simulink model "WaterTank"  (R2025b)
settings: Solver=ode4  StartTime=0.0  StopTime=60  FixedStep=0.01  RelTol=1e-3
InitFcn:
  | WaterTank_script;
undefined symbols (not defined in the file or in its folder): DiscIntNeverNeededParam
libraries: simulink x3, slpidlib x1, rllib x1
settings Model: Creator=Administrator  LastModifiedBy=chang

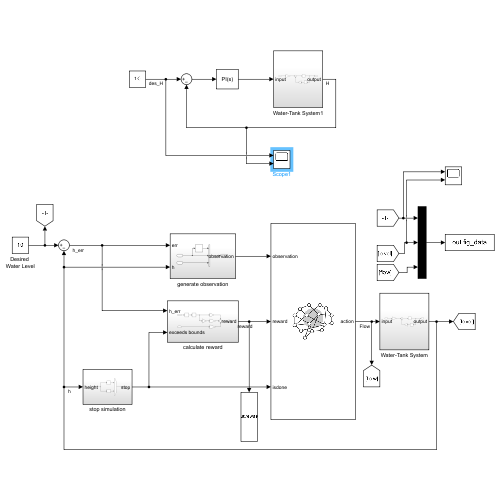
[thumbnail: Simulink's stored preview of the top-level diagram]
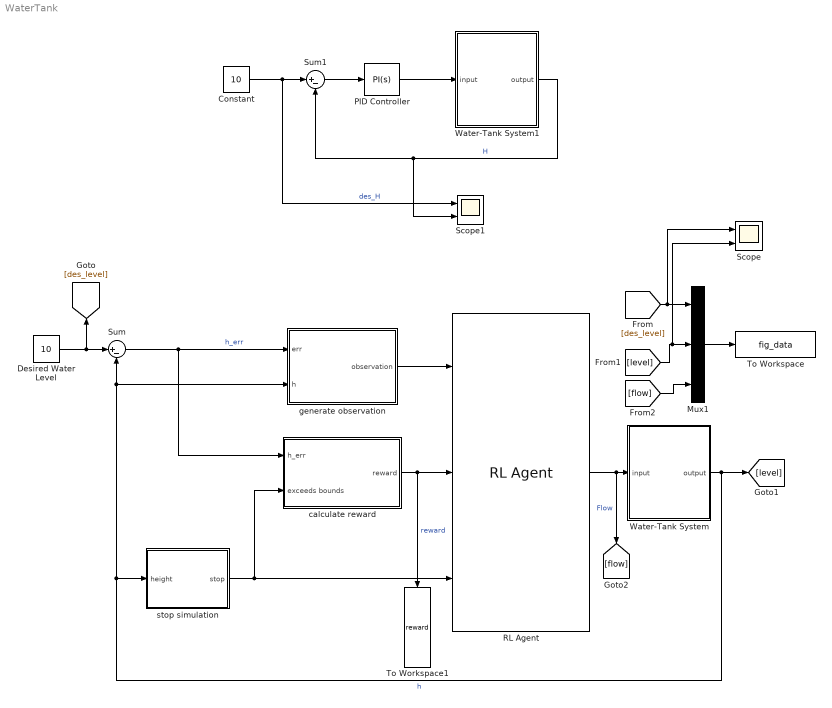
== system WaterTank ==
  Constant : Constant  Value=10
  Desired Water Level : Constant  Value=10
  Mux1 : Mux  Inputs=3
  PID Controller : slpidlib/PID Controller  Controller=PI  Form=Parallel  TimeDomain=Continuous-time  UseExternalTs=off  SampleTime=-1  IntegratorMethod=Forward Euler  FilterMethod=Forward Euler  ControllerParametersSource=internal  P=1.5  I=0.07  UseKiTs=off  D=0  UseExternalDerivativeSource=off  N=100  UseFilter=on  TunerSelectOption=Transfer Function Based (PID Tuner App)  InitialConditionSource=internal  InitialConditionForIntegrator=0  InitialConditionForFilter=0  DifferentiatorICPrevScaledInput=0  ExternalReset=none  TrackingMode=off  Kt=1  LimitOutput=off  SatLimitsSource=internal  UpperSaturationLimit=inf  LowerSaturationLimit=-inf  LinearizeAsGain=on  AntiWindupMode=none  Kb=1  LimitIntegrator=off  UpperIntegratorSaturationLimit=inf  LowerIntegratorSaturationLimit=-inf  POutMin=[]  POutMax=[]  IOutMin=[]  IOutMax=[]  DOutMin=[]  DOutMax=[]  NOutMin=[]  NOutMax=[]  SumOutMin=[]  SumOutMax=[]  SaturationOutMin=[]  SaturationOutMax=[]  PParamMin=[]  PParamMax=[]  IParamMin=[]  IParamMax=[]  DParamMin=[]  DParamMax=[]  NParamMin=[]  NParamMax=[]  KbParamMin=[]  KbParamMax=[]  KtParamMin=[]  KtParamMax=[]  KbOutMin=[]  KbOutMax=[]  KtOutMin=[]  KtOutMax=[]  IntegratorOutMin=[]  IntegratorOutMax=[]  FilterOutMin=[]  FilterOutMax=[]  SumI1OutMin=[]  SumI1OutMax=[]  SumI2OutMin=[]  SumI2OutMax=[]  SumI3OutMin=[]  SumI3OutMax=[]  SumI4OutMin=[]  SumI4OutMax=[]  SumDOutMin=[]  SumDOutMax=[]  DifferentiatorOutMin=[]  DifferentiatorOutMax=[]  FilterDiffOutCoefMin=[]  FilterDiffOutCoefMax=[]  ReciprocalOutMin=[]  ReciprocalOutMax=[]  SumDenOutMin=[]  SumDenOutMax=[]  SumNumOutMin=[]  SumNumOutMax=[]  DivideOutMin=[]  DivideOutMax=[]  UdiffTsProdOutMin=[]  UdiffTsProdOutMax=[]  NTsProdOutMin=[]  NTsProdOutMax=[]  UintegralTsProdOutMin=[]  UintegralTsProdOutMax=[]  UngainTsProdOutMin=[]  UngainTsProdOutMax=[]  ClampingZeroOutDataTypeStr=Inherit: Inherit via back propagation  ClampingZeroOutMin=[]  ClampingZeroOutMax=[]  FilterDenConstantOutDataTypeStr=Inherit: Inherit via back propagation  FilterDenConstantOutMin=[]  FilterDenConstantOutMax=[]  PCopyOutDataTypeStr=Inherit: Inherit via back propagation  PCopyOutMin=[]  PCopyOutMax=[]  NCopyOutDataTypeStr=Inherit: Inherit via back propagation  NCopyOutMin=[]  NCopyOutMax=[]  IntegratorContinuousStateAttributes=''  IntegratorStateMustResolveToSignalObject=off  IntegratorRTWStateStorageClass=Auto  FilterContinuousStateAttributes=''  FilterStateMustResolveToSignalObject=off  FilterRTWStateStorageClass=Auto  ParallelPVariant=InternalParameters  IdealPVariant=Disabled  IVariant=InternalParameters  DVariant=Disabled  IntegratorVariant=Continuous  SatVariant=Disabled  AWVariant=Passthrough  PCopyVariant=Disabled  TRVariant=Disabled  FdbkBlocksVariant=Forward  IdealPFdbkVariant=Disabled  SatFdbkVariant=Disabled  DerivativeFilterVariant=Disabled  NVariant=Disabled  NCopyVariant=Disabled_SignalSpec  FilterICVariant=Disabled  IntegratorICVariant=InternalICs  ExternalResetVariant=Disabled  TRSumVariant=Passthrough  SumFdbkVariant=Disabled  SumVariant=Sum_PI  TsampFilterVariant=InternalTs  TsampNgainVariant=Passthrough  TsampIntegralVariant=Disabled_SignalSpec  ExternalSaturationOutDataTypeStr=Inherit: Same as second input  DerivativeSourceVariant=Disabled  PreIntVariant=InternalPreInt
  RL Agent : rllib/RL Agent  Agent=agent  ExternalActionAsInput=off  ProvideLastAction=off  ProvideCumRwd=off  TreatAsDirectFeedthrough=on  UseStrictObservationDataTypes=off
  Scope : Scope  NumInputPorts=2
      settings: ShowGrid=off  ActiveDisplayYMinimum=2.1234199736626467  ActiveDisplayYMaximum=10.889220237036184  YLabel=높이 (m)
  Scope1 : Scope  NumInputPorts=2
      settings: ShowGrid=off  ActiveDisplayYMinimum=2.1193690493953312  ActiveDisplayYMaximum=10.925678555442021  YLabel=높이 (m)
  Sum : Sum  Inputs=|+-
  Sum1 : Sum  Inputs=|+-
  To Workspace : ToWorkspace  VariableName=fig_data  SaveFormat=Timeseries  SampleTime=-1
  To Workspace1 : ToWorkspace  VariableName=reward  SaveFormat=Timeseries  SampleTime=-1
  Water-Tank System : Subsystem
  Water-Tank System1 : Subsystem
  calculate reward : Subsystem
  generate observation : Subsystem
  stop simulation : Subsystem
  wires:
  Water-Tank System/1(output) -> [level], generate observation/2(h), Sum/2, stop simulation/1(height)  "h"
  stop simulation/1(stop) -> calculate reward/2(exceeds bounds), RL Agent/3
  calculate reward/1(reward) -> RL Agent/2, To Workspace1/1  "reward"
  RL Agent/1 -> [flow], Water-Tank System/1(input)  "Flow"
  Desired Water Level/1 -> [des_level], Sum/1
  [des_level] -> Scope/1, Mux1/1
  [level] -> Scope/2, Mux1/2
  [flow] -> Mux1/3
  Sum/1 -> calculate reward/1(h_err), generate observation/1(err)  "h_err"
  generate observation/1(observation) -> RL Agent/1
  Mux1/1 -> To Workspace/1
  Constant/1 -> Scope1/1, Sum1/1  "des_H"
  Sum1/1 -> PID Controller/1
  PID Controller/1 -> Water-Tank System1/1(input)
  Water-Tank System1/1(output) -> Scope1/2, Sum1/2  "H"

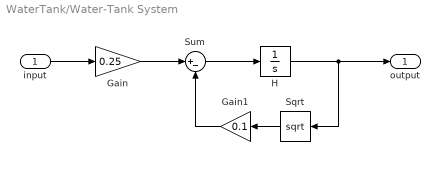
== system WaterTank/Water-Tank System ==
  input : Inport
  Gain : Gain  Gain=0.25
  Gain1 : Gain  Gain=0.1
  H : Integrator  InitialCondition=3  LimitOutput=on  LowerSaturationLimit=0
  Sqrt : Sqrt  OutputSignalType=real
  Sum : Sum  Inputs=|+-
  output : Outport
  wires:
  input/1 -> Gain/1
  Sum/1 -> H/1
  H/1 -> Sqrt/1, output/1
  Gain/1 -> Sum/1
  Sqrt/1 -> Gain1/1
  Gain1/1 -> Sum/2

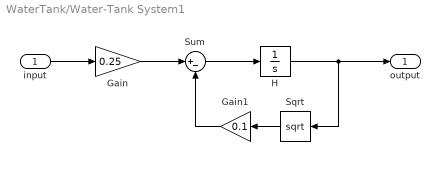
== system WaterTank/Water-Tank System1 ==
  input : Inport
  Gain : Gain  Gain=0.25
  Gain1 : Gain  Gain=0.1
  H : Integrator  InitialCondition=3  LimitOutput=on  LowerSaturationLimit=0
  Sqrt : Sqrt  OutputSignalType=real
  Sum : Sum  Inputs=|+-
  output : Outport
  wires:
  input/1 -> Gain/1
  Sum/1 -> H/1
  H/1 -> Sqrt/1, output/1
  Gain/1 -> Sum/1
  Sqrt/1 -> Gain1/1
  Gain1/1 -> Sum/2

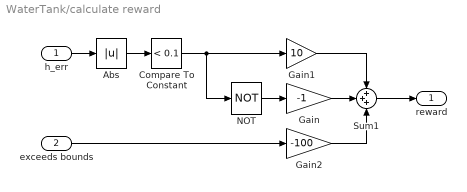
== system WaterTank/calculate reward ==
  h_err : Inport
  exceeds bounds : Inport  Port=2
  Abs : Abs  SaturateOnIntegerOverflow=off
  Compare To Constant : simulink/Logic and Bit Operations/Compare To Constant  relop=<  const=0.1  OutDataTypeStr=boolean
  Gain : Gain  Gain=-1
  Gain1 : Gain  Gain=10
  Gain2 : Gain  Gain=-100
  NOT : Logic  Operator=NOT  IconShape=distinctive  AllPortsSameDT=off  OutDataTypeStr=boolean
  Sum1 : Sum  Inputs=+++
  reward : Outport
  wires:
  Sum1/1 -> reward/1
  Gain2/1 -> Sum1/3
  NOT/1 -> Gain/1
  h_err/1 -> Abs/1
  Compare To Constant/1 -> Gain1/1, NOT/1
  Gain/1 -> Sum1/2
  exceeds bounds/1 -> Gain2/1
  Gain1/1 -> Sum1/1
  Abs/1 -> Compare To Constant/1

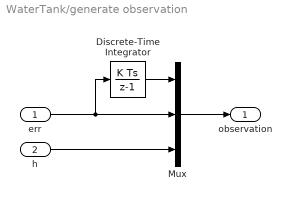
== system WaterTank/generate observation ==
  err : Inport
  h : Inport  Port=2
  Discrete-Time Integrator : DiscreteIntegrator  SampleTime=1.0  ICPrevOutput=DiscIntNeverNeededParam  ICPrevScaledInput=DiscIntNeverNeededParam
  Mux : Mux  Inputs=3
  observation : Outport
  wires:
  Discrete-Time Integrator/1 -> Mux/1
  h/1 -> Mux/3
  Mux/1 -> observation/1
  err/1 -> Discrete-Time Integrator/1, Mux/2

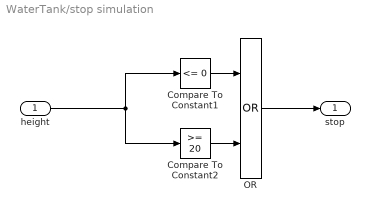
== system WaterTank/stop simulation ==
  height : Inport
  Compare To Constant1 : simulink/Logic and Bit Operations/Compare To Constant  relop=<=  const=0  OutDataTypeStr=boolean
  Compare To Constant2 : simulink/Logic and Bit Operations/Compare To Constant  relop=>=  const=20  OutDataTypeStr=boolean
  OR : Logic  Operator=OR  IconShape=distinctive  AllPortsSameDT=off  OutDataTypeStr=boolean
  stop : Outport
  wires:
  Compare To Constant1/1 -> OR/1
  height/1 -> Compare To Constant2/1, Compare To Constant1/1
  Compare To Constant2/1 -> OR/2
  OR/1 -> stop/1
